simulink model "t_wit_sim_w_motor_model"  (R2014a)
settings: Solver=ode45  StartTime=0.0  StopTime=6  RelTol=1e-3
values from neighbouring files (symbols this model uses):
  A_r = [0 1;0 0]    [T_WIT.m]    (also in t_wit_w_motor_model.m)
  A_t = zeros(4,4)    [T_WIT.m]    (also in t_wit_w_motor_model.m)
  B_r = [0;6/((9*Mr+Mp)*R*D)]    [T_WIT.m]    (also in t_wit_w_motor_model.m)
  B_t = zeros(4,1)    [T_WIT.m]    (also in t_wit_w_motor_model.m)
  C_r = eye(2)    [T_WIT.m]    (also in t_wit_w_motor_model.m)
  C_t = eye(4)    [T_WIT.m]    (also in t_wit_w_motor_model.m)
  D_r = zeros(2,1)    [T_WIT.m]    (also in t_wit_w_motor_model.m)
  D_t = zeros(4,1)    [T_WIT.m]    (also in t_wit_w_motor_model.m)
  Den = [J*L_m (J*R_m+L_m*B) (B*R_m+K_m^2)]    [t_wit_w_motor_model.m]
  J = 0.0188    [t_wit_w_motor_model.m]
  K1 = lqr(A_t,B_t,Q,R)    [T_WIT.m]    (also in t_wit_w_motor_model.m = place(A_t,B_t,p1))
  K2 = place(A_r,B_r,p2)    [T_WIT.m]    (also in t_wit_w_motor_model.m)
  K_i = 0    [t_wit_w_motor_model.m]
  K_m = 1.082    [t_wit_w_motor_model.m]
  K_p = 1.65    [t_wit_w_motor_model.m]
  Psi_dot_in = 0*(pi/180)    (= 0)    [T_WIT.m]    (also in t_wit_w_motor_model.m)
  Theta_d = 5*(pi/180)    (= 0.0872664625997)    [T_WIT.m]    (also in t_wit_w_motor_model.m = 0.523598775598)
  V_in = 0.00    (= 0)    [T_WIT.m]    (also in t_wit_w_motor_model.m)
libraries: simulink x2
settings Model: Creator=jeson_000  LastModifiedBy=jeson_000

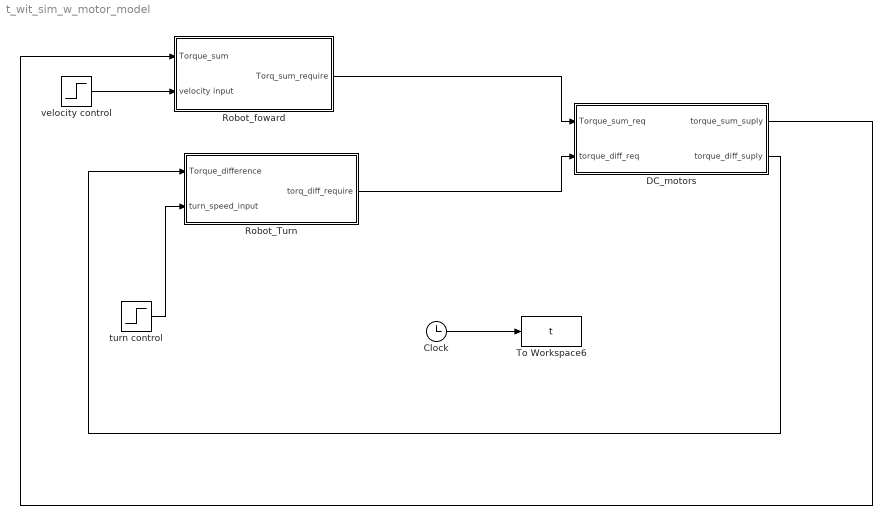
== system t_wit_sim_w_motor_model ==
  Clock : Clock
  DC_motors : Subsystem
  Robot_Turn : Subsystem
  Robot_foward : Subsystem
  To Workspace6 : ToWorkspace  VariableName=t  SampleTime=-1
  turn control : Step  After=Psi_dot_in  SampleTime=0
  velocity control : Step  After=V_in  SampleTime=0
  wires:
  Clock/1 -> To Workspace6/1
  velocity control/1 -> Robot_foward/2(velocity input)
  turn control/1 -> Robot_Turn/2(turn_speed_input)
  DC_motors/1(torque_sum_suply) -> Robot_foward/1(Torque_sum)
  DC_motors/2(torque_diff_suply) -> Robot_Turn/1(Torque_difference)
  Robot_foward/1(Torq_sum_require) -> DC_motors/1(Torque_sum_req)
  Robot_Turn/1(torq_diff_require) -> DC_motors/2(torque_diff_req)

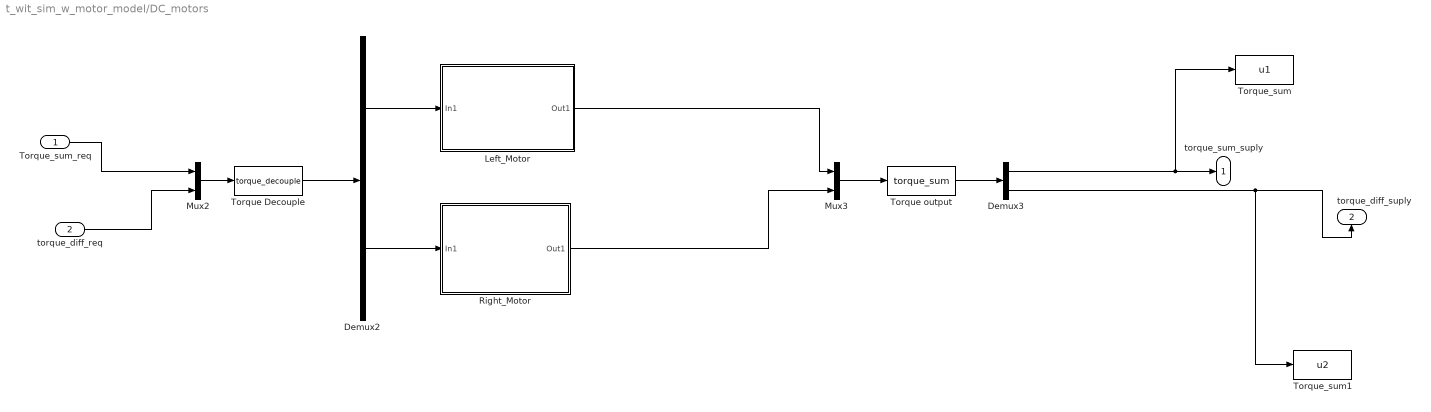
== system t_wit_sim_w_motor_model/DC_motors ==
  Torque_sum_req : Inport
  torque_diff_req : Inport  Port=2
  Demux2 : Demux  Outputs=2
  Demux3 : Demux  Outputs=2
  Left_Motor : Subsystem
  Mux2 : Mux  Inputs=2
  Mux3 : Mux  Inputs=2
  Right_Motor : Subsystem
  Torque Decouple : MATLABFcn  MATLABFcn=torque_decouple  OutputDimensions=2
  Torque output : MATLABFcn  MATLABFcn=torque_sum  OutputDimensions=2
  Torque_sum : ToWorkspace  VariableName=u1  SampleTime=-1
  Torque_sum1 : ToWorkspace  VariableName=u2  SampleTime=-1
  torque_sum_suply : Outport
  torque_diff_suply : Outport  Port=2
  wires:
  torque_diff_req/1 -> Mux2/2
  Mux2/1 -> Torque Decouple/1
  Torque Decouple/1 -> Demux2/1
  Demux3/2 -> Torque_sum1/1, torque_diff_suply/1
  Demux3/1 -> Torque_sum/1, torque_sum_suply/1
  Torque output/1 -> Demux3/1
  Mux3/1 -> Torque output/1
  Torque_sum_req/1 -> Mux2/1
  Demux2/1 -> Left_Motor/1(In1)
  Left_Motor/1(Out1) -> Mux3/1
  Demux2/2 -> Right_Motor/1(In1)
  Right_Motor/1(Out1) -> Mux3/2

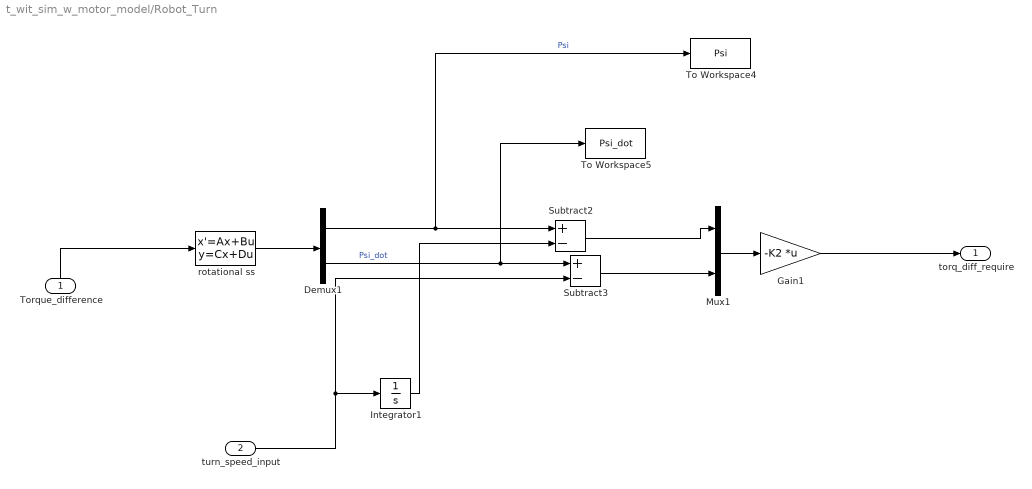
== system t_wit_sim_w_motor_model/Robot_Turn ==
  Torque_difference : Inport
  turn_speed_input : Inport  Port=2
  Demux1 : Demux  Outputs=2
  Gain1 : Gain  Gain=-K2  Multiplication=Matrix(K*u)
  Integrator1 : Integrator
  Mux1 : Mux  Inputs=2
  Subtract2 : Sum  Inputs=+-
  Subtract3 : Sum  Inputs=+-
  To Workspace4 : ToWorkspace  VariableName=Psi  SampleTime=-1
  To Workspace5 : ToWorkspace  VariableName=Psi_dot  SampleTime=-1
  rotational ss : StateSpace  A=A_r  B=B_r  C=C_r  D=D_r  X0=0
  torq_diff_require : Outport
  wires:
  Torque_difference/1 -> rotational ss/1
  Gain1/1 -> torq_diff_require/1
  turn_speed_input/1 -> Subtract3/2, Integrator1/1
  Subtract2/1 -> Mux1/1
  rotational ss/1 -> Demux1/1
  Demux1/1 -> To Workspace4/1, Subtract2/1  "Psi"
  Mux1/1 -> Gain1/1
  Integrator1/1 -> Subtract2/2
  Demux1/2 -> To Workspace5/1, Subtract3/1  "Psi_dot"
  Subtract3/1 -> Mux1/2

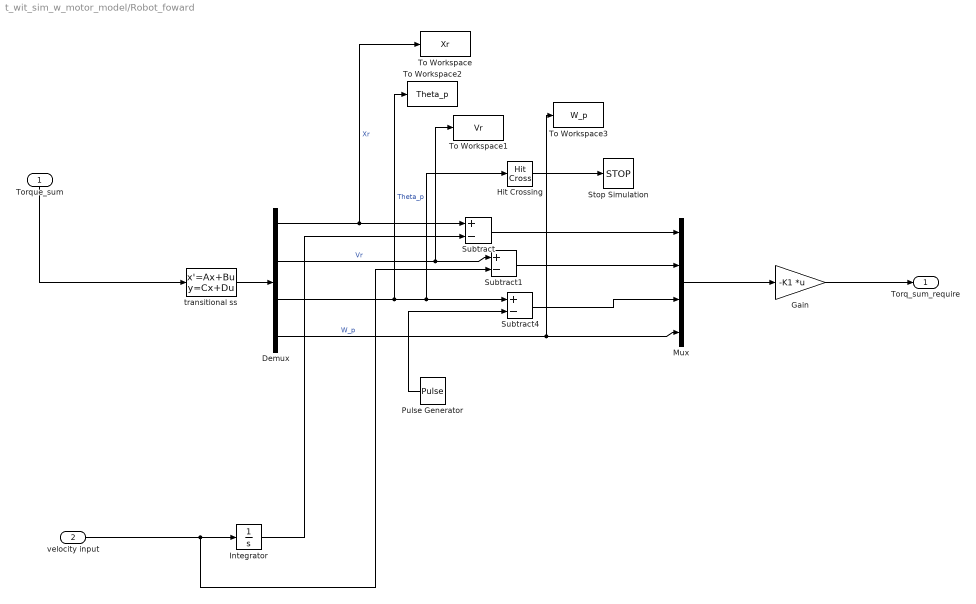
== system t_wit_sim_w_motor_model/Robot_foward ==
  Torque_sum : Inport
  velocity input : Inport  Port=2
  Demux : Demux
  Gain : Gain  Gain=-K1  Multiplication=Matrix(K*u)
  Hit Crossing : HitCross  HitCrossingOffset=-pi/2
  Integrator : Integrator
  Mux : Mux
  Pulse Generator : DiscretePulseGenerator  PulseType=Time based  Amplitude=Theta_d  Period=10
  Stop Simulation : Stop
  Subtract : Sum  Inputs=+-
  Subtract1 : Sum  Inputs=+-
  Subtract4 : Sum  Inputs=+-
  To Workspace : ToWorkspace  VariableName=Xr  SampleTime=-1
  To Workspace1 : ToWorkspace  VariableName=Vr  SampleTime=-1
  To Workspace2 : ToWorkspace  VariableName=Theta_p  SampleTime=-1
  To Workspace3 : ToWorkspace  VariableName=W_p  SampleTime=-1
  transitional ss : StateSpace  A=A_t  B=B_t  C=C_t  D=D_t  X0=0
  Torq_sum_require : Outport
  wires:
  Subtract/1 -> Mux/1
  Gain/1 -> Torq_sum_require/1
  Demux/4 -> To Workspace3/1, Mux/4  "W_p"
  Integrator/1 -> Subtract/2
  Pulse Generator/1 -> Subtract4/2
  Subtract4/1 -> Mux/3
  Demux/1 -> Subtract/1, To Workspace/1  "Xr"
  Demux/2 -> To Workspace1/1, Subtract1/1  "Vr"
  transitional ss/1 -> Demux/1
  Demux/3 -> Subtract4/1, Hit Crossing/1, To Workspace2/1  "Theta_p"
  Subtract1/1 -> Mux/2
  Hit Crossing/1 -> Stop Simulation/1
  velocity input/1 -> Subtract1/2, Integrator/1
  Mux/1 -> Gain/1
  Torque_sum/1 -> transitional ss/1

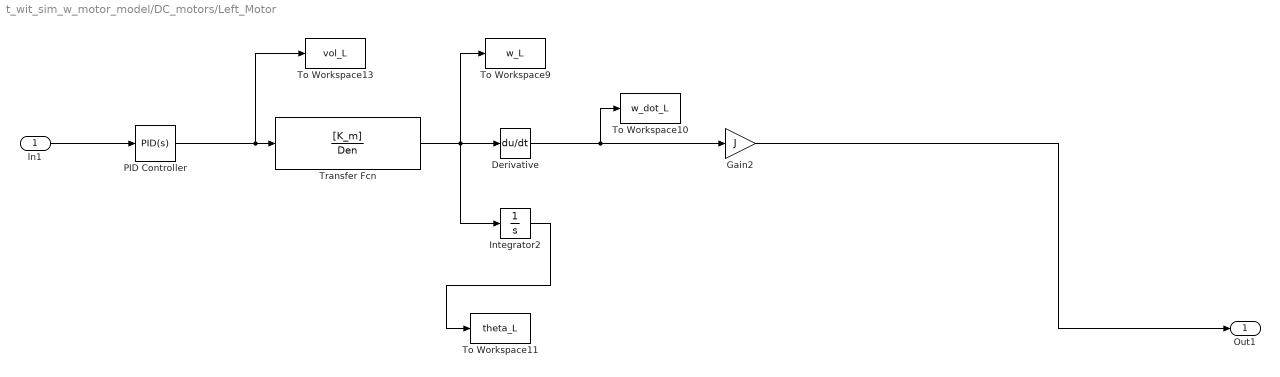
== system t_wit_sim_w_motor_model/DC_motors/Left_Motor ==
  In1 : Inport
  Derivative : Derivative
  Gain2 : Gain  Gain=J
  Integrator2 : Integrator
  PID Controller : simulink/Continuous/PID Controller  Controller=PID  TimeDomain=Continuous-time  SampleTime=1  IntegratorMethod=Forward Euler  FilterMethod=Forward Euler  Form=Parallel  P=K_p  I=K_i  D=0  N=100  InitialConditionSource=internal  InitialConditionForIntegrator=0  InitialConditionForFilter=0  ExternalReset=none  LimitOutput=off  UpperSaturationLimit=inf  LowerSaturationLimit=-inf  LinearizeAsGain=on  AntiWindupMode=none  Kb=1  TrackingMode=off  Kt=1  PParamMin=[]  PParamMax=[]  IParamMin=[]  IParamMax=[]  DParamMin=[]  DParamMax=[]  NParamMin=[]  NParamMax=[]  KbParamMin=[]  KbParamMax=[]  KtParamMin=[]  KtParamMax=[]  POutMin=[]  POutMax=[]  IOutMin=[]  IOutMax=[]  DOutMin=[]  DOutMax=[]  NOutMin=[]  NOutMax=[]  KbOutMin=[]  KbOutMax=[]  KtOutMin=[]  KtOutMax=[]  IntegratorOutMin=[]  IntegratorOutMax=[]  FilterOutMin=[]  FilterOutMax=[]  SumOutMin=[]  SumOutMax=[]  SumI1OutMin=[]  SumI1OutMax=[]  SumI2OutMin=[]  SumI2OutMax=[]  SumI3OutMin=[]  SumI3OutMax=[]  SumDOutMin=[]  SumDOutMax=[]  SaturationOutMin=[]  SaturationOutMax=[]  IntegratorContinuousStateAttributes=''  IntegratorStateMustResolveToSignalObject=off  IntegratorRTWStateStorageClass=Auto  FilterContinuousStateAttributes=''  FilterStateMustResolveToSignalObject=off  FilterRTWStateStorageClass=Auto
  To Workspace10 : ToWorkspace  VariableName=w_dot_L  SampleTime=-1
  To Workspace11 : ToWorkspace  VariableName=theta_L  SampleTime=-1
  To Workspace13 : ToWorkspace  VariableName=vol_L  SampleTime=-1
  To Workspace9 : ToWorkspace  VariableName=w_L  SampleTime=-1
  Transfer Fcn : TransferFcn  Numerator=[K_m]  Denominator=Den
  Out1 : Outport
  wires:
  In1/1 -> PID Controller/1
  Gain2/1 -> Out1/1
  Transfer Fcn/1 -> Integrator2/1, Derivative/1, To Workspace9/1
  PID Controller/1 -> To Workspace13/1, Transfer Fcn/1
  Derivative/1 -> Gain2/1, To Workspace10/1
  Integrator2/1 -> To Workspace11/1

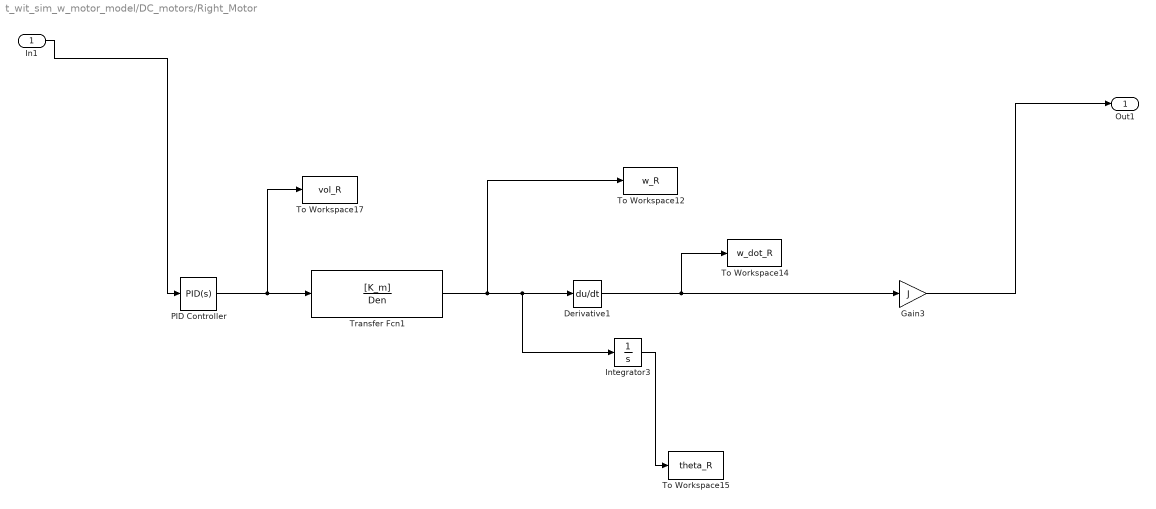
== system t_wit_sim_w_motor_model/DC_motors/Right_Motor ==
  In1 : Inport
  Derivative1 : Derivative
  Gain3 : Gain  Gain=J
  Integrator3 : Integrator
  PID Controller : simulink/Continuous/PID Controller  Controller=PID  TimeDomain=Continuous-time  SampleTime=1  IntegratorMethod=Forward Euler  FilterMethod=Forward Euler  Form=Parallel  P=K_p  I=K_i  D=0  N=100  InitialConditionSource=internal  InitialConditionForIntegrator=0  InitialConditionForFilter=0  ExternalReset=none  LimitOutput=off  UpperSaturationLimit=inf  LowerSaturationLimit=-inf  LinearizeAsGain=on  AntiWindupMode=none  Kb=1  TrackingMode=off  Kt=1  PParamMin=[]  PParamMax=[]  IParamMin=[]  IParamMax=[]  DParamMin=[]  DParamMax=[]  NParamMin=[]  NParamMax=[]  KbParamMin=[]  KbParamMax=[]  KtParamMin=[]  KtParamMax=[]  POutMin=[]  POutMax=[]  IOutMin=[]  IOutMax=[]  DOutMin=[]  DOutMax=[]  NOutMin=[]  NOutMax=[]  KbOutMin=[]  KbOutMax=[]  KtOutMin=[]  KtOutMax=[]  IntegratorOutMin=[]  IntegratorOutMax=[]  FilterOutMin=[]  FilterOutMax=[]  SumOutMin=[]  SumOutMax=[]  SumI1OutMin=[]  SumI1OutMax=[]  SumI2OutMin=[]  SumI2OutMax=[]  SumI3OutMin=[]  SumI3OutMax=[]  SumDOutMin=[]  SumDOutMax=[]  SaturationOutMin=[]  SaturationOutMax=[]  IntegratorContinuousStateAttributes=''  IntegratorStateMustResolveToSignalObject=off  IntegratorRTWStateStorageClass=Auto  FilterContinuousStateAttributes=''  FilterStateMustResolveToSignalObject=off  FilterRTWStateStorageClass=Auto
  To Workspace12 : ToWorkspace  VariableName=w_R  SampleTime=-1
  To Workspace14 : ToWorkspace  VariableName=w_dot_R  SampleTime=-1
  To Workspace15 : ToWorkspace  VariableName=theta_R  SampleTime=-1
  To Workspace17 : ToWorkspace  VariableName=vol_R  SampleTime=-1
  Transfer Fcn1 : TransferFcn  Numerator=[K_m]  Denominator=Den
  Out1 : Outport
  wires:
  Derivative1/1 -> Gain3/1, To Workspace14/1
  Gain3/1 -> Out1/1
  Transfer Fcn1/1 -> Derivative1/1, Integrator3/1, To Workspace12/1
  In1/1 -> PID Controller/1
  Integrator3/1 -> To Workspace15/1
  PID Controller/1 -> Transfer Fcn1/1, To Workspace17/1
